simulink model "Single_phase_PF_measurement"  (R2024a)
settings: Solver=ode23  StartTime=0.0  StopTime=0.1  RelTol=1e-4
libraries: spsACVoltageSourceLib x3, spsCurrentMeasurementLib x3, spsPowerLib x3, spsSeriesRLCBranchLib x3, spsVoltageMeasurementLib x3, spspowerguiLib x3, spsRMSLib x2
settings Model: Creator=User  LastModifiedBy=User

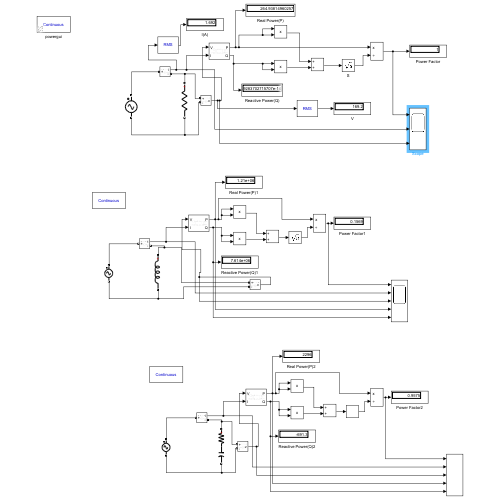
[thumbnail: Simulink's stored preview of the top-level diagram]
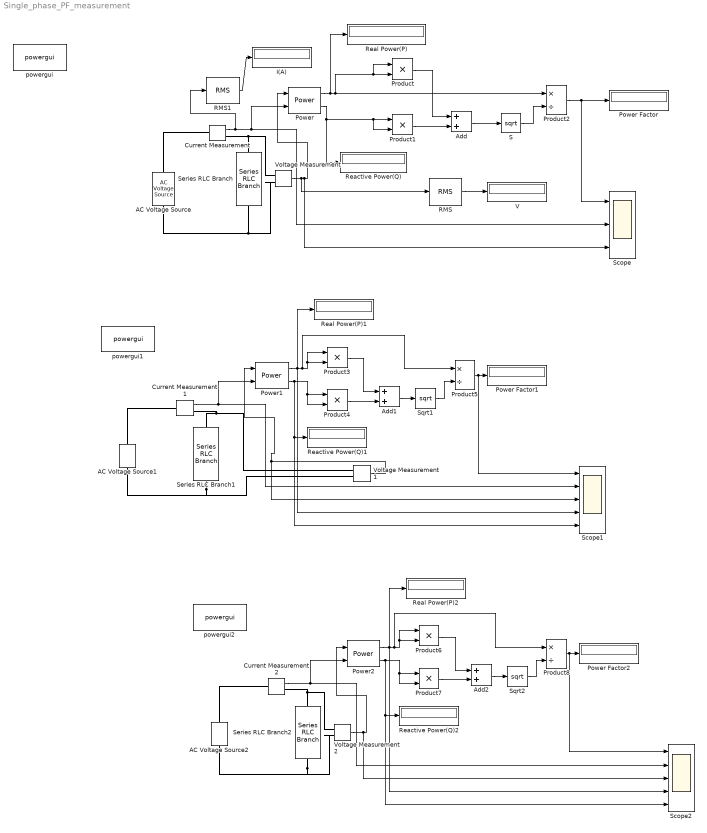
== system Single_phase_PF_measurement ==
  AC Voltage Source : spsACVoltageSourceLib/AC Voltage Source  Amplitude=230  Phase=0  Frequency=50  SampleTime=0  Measurements=None  BusType=swing  Pref=10e3  Qref=0  Qmin=-inf  Qmax=+inf
  AC Voltage Source1 : spsACVoltageSourceLib/AC Voltage Source  Amplitude=230  Phase=0  Frequency=50  SampleTime=0  Measurements=None  BusType=swing  Pref=10e3  Qref=0  Qmin=-inf  Qmax=+inf
  AC Voltage Source2 : spsACVoltageSourceLib/AC Voltage Source  Amplitude=230  Phase=0  Frequency=50  SampleTime=0  Measurements=None  BusType=swing  Pref=10e3  Qref=0  Qmin=-inf  Qmax=+inf
  Add : Sum
  Add1 : Sum
  Add2 : Sum
  Current Measurement : spsCurrentMeasurementLib/Current Measurement  PhasorSimulation=off  OutputType=Complex  PSBequivalent=0
  Current Measurement1 : spsCurrentMeasurementLib/Current Measurement  PhasorSimulation=off  OutputType=Complex  PSBequivalent=0
  Current Measurement2 : spsCurrentMeasurementLib/Current Measurement  PhasorSimulation=off  OutputType=Complex  PSBequivalent=0
  I(A) : Display
  Power : spsPowerLib/Power  Freq=60  Vinit=[1, 0]  Iinit=[1, 0]  Ts=0
  Power Factor : Display
  Power Factor1 : Display
  Power Factor2 : Display
  Power1 : spsPowerLib/Power  Freq=60  Vinit=[1, 0]  Iinit=[1, 0]  Ts=0
  Power2 : spsPowerLib/Power  Freq=60  Vinit=[1, 0]  Iinit=[1, 0]  Ts=0
  Product{,1,3..4,6..7} (6 alike) : Product
  Product2 : Product  Inputs=*/
  Product5 : Product  Inputs=*/
  Product8 : Product  Inputs=*/
  RMS : spsRMSLib/RMS  TrueRMS=on  Freq=60  RMSInit=120  Ts=0
  RMS1 : spsRMSLib/RMS  TrueRMS=on  Freq=60  RMSInit=120  Ts=0
  Reactive Power(Q) : Display
  Reactive Power(Q)1 : Display
  Reactive Power(Q)2 : Display
  Real Power(P) : Display
  Real Power(P)1 : Display
  Real Power(P)2 : Display
  S : Sqrt
  Scope : Scope  NumInputPorts=3
  Scope1 : Scope  NumInputPorts=5
  Scope2 : Scope  NumInputPorts=5
  Series RLC Branch : spsSeriesRLCBranchLib/Series RLC Branch  LConnTagsString=__new0  RConnTagsString=__new0  BranchType=R  Resistance=100  Inductance=1  SetiL0=off  InitialCurrent=0  Capacitance=40e-6  Setx0=off  InitialVoltage=0  Measurements=None
  Series RLC Branch1 : spsSeriesRLCBranchLib/Series RLC Branch  LConnTagsString=__new0  RConnTagsString=__new0  BranchType=L  Resistance=10  Inductance=10e-6  SetiL0=off  InitialCurrent=0  Capacitance=1e-6  Setx0=off  InitialVoltage=0  Measurements=None
  Series RLC Branch2 : spsSeriesRLCBranchLib/Series RLC Branch  LConnTagsString=__new0  RConnTagsString=__new0  BranchType=RC  Resistance=10  Inductance=10e-6  SetiL0=off  InitialCurrent=0  Capacitance=1e-3  Setx0=off  InitialVoltage=0  Measurements=None
  Sqrt1 : Sqrt
  Sqrt2 : Sqrt
  V : Display
  Voltage Measurement : spsVoltageMeasurementLib/Voltage Measurement  PhasorSimulation=off  OutputType=Complex  PSBequivalent=0
  Voltage Measurement1 : spsVoltageMeasurementLib/Voltage Measurement  PhasorSimulation=off  OutputType=Complex  PSBequivalent=0
  Voltage Measurement2 : spsVoltageMeasurementLib/Voltage Measurement  PhasorSimulation=off  OutputType=Complex  PSBequivalent=0
  powergui : spspowerguiLib/powergui  Priority=1  SimulationMode=Continuous  SampleTime=50e-6  frequency=60  Iterations=50  frequencyindice=50  Pbase=100e6  ErrMax=1e-4  UnitsV=kV  UnitsW=MW  buscounter=0  FunctionMessages=off  echomessages=off  EnableUseOfTLC=off  CurrentSourceSwitches=off  DisableSnubberDevices=off  DisableRonSwitches=off  DisableVfSwitches=off  DisplayEquations=off  AutomaticDiscreteSolvers=off  SolverType=Tustin/Backward Euler (TBE)  Interpol=off  ExternalGateDelay=off  methode=off  Ts=100  x0status=blocks  SPID=on  SwTol=0  HookPort=off  NonlinearTolerance=1e-4  nMaxIteration=100  ContinueOnMaxIteration=off  RestoreLinks=warning  ResistiveCurrentMeasurement=off  Frange=[0:2:500]  Ylog=off  Xlog=on  ShowGrid=off  save=off  variable=ZData  structure=0  ZoomFFT=off  StartTime=0.0  cycles=1  DisplayStyle=1  fundamental=60  FreqAxis=off  MaxFrequency=1000  frequencyindicesteady=1  RmsSteady=1  display=off
  powergui1 : spspowerguiLib/powergui  Priority=1  SimulationMode=Continuous  SampleTime=50e-6  frequency=60  Iterations=50  frequencyindice=50  Pbase=100e6  ErrMax=1e-4  UnitsV=kV  UnitsW=MW  buscounter=0  FunctionMessages=off  echomessages=off  EnableUseOfTLC=off  CurrentSourceSwitches=off  DisableSnubberDevices=off  DisableRonSwitches=off  DisableVfSwitches=off  DisplayEquations=off  AutomaticDiscreteSolvers=off  SolverType=Tustin/Backward Euler (TBE)  Interpol=off  ExternalGateDelay=off  methode=off  Ts=100  x0status=blocks  SPID=on  SwTol=0  HookPort=off  NonlinearTolerance=1e-4  nMaxIteration=100  ContinueOnMaxIteration=off  RestoreLinks=warning  ResistiveCurrentMeasurement=off  Frange=[0:2:500]  Ylog=off  Xlog=on  ShowGrid=off  save=off  variable=ZData  structure=0  ZoomFFT=off  StartTime=0.0  cycles=1  DisplayStyle=1  fundamental=60  FreqAxis=off  MaxFrequency=1000  frequencyindicesteady=1  RmsSteady=1  display=off
  powergui2 : spspowerguiLib/powergui  Priority=1  SimulationMode=Continuous  SampleTime=50e-6  frequency=60  Iterations=50  frequencyindice=50  Pbase=100e6  ErrMax=1e-4  UnitsV=kV  UnitsW=MW  buscounter=0  FunctionMessages=off  echomessages=off  EnableUseOfTLC=off  CurrentSourceSwitches=off  DisableSnubberDevices=off  DisableRonSwitches=off  DisableVfSwitches=off  DisplayEquations=off  AutomaticDiscreteSolvers=off  SolverType=Tustin/Backward Euler (TBE)  Interpol=off  ExternalGateDelay=off  methode=off  Ts=100  x0status=blocks  SPID=on  SwTol=0  HookPort=off  NonlinearTolerance=1e-4  nMaxIteration=100  ContinueOnMaxIteration=off  RestoreLinks=warning  ResistiveCurrentMeasurement=off  Frange=[0:2:500]  Ylog=off  Xlog=on  ShowGrid=off  save=off  variable=ZData  structure=0  ZoomFFT=off  StartTime=0.0  cycles=1  DisplayStyle=1  fundamental=60  FreqAxis=off  MaxFrequency=1000  frequencyindicesteady=1  RmsSteady=1  display=off
  wires:
  Voltage Measurement/1 -> RMS/1, Scope/3, Power/1
  Current Measurement/1 -> RMS1/1, Power/2, Scope/2
  Power/1 -> Real Power(P)/1, Product2/1, Product/2, Product/1
  Power/2 -> Reactive Power(Q)/1, Product1/2, Product1/1
  Add/1 -> S/1
  Product/1 -> Add/1
  Product1/1 -> Add/2
  S/1 -> Product2/2
  Product2/1 -> Scope/1, Power Factor/1
  Add1/1 -> Sqrt1/1
  Sqrt1/1 -> Product5/2
  Power1/2 -> Scope1/5, Reactive Power(Q)1/1, Product4/2, Product4/1
  Current Measurement1/1 -> Scope1/2, Power1/2
  Voltage Measurement1/1 -> Scope1/3, Power1/1
  Product5/1 -> Scope1/1, Power Factor1/1
  Product4/1 -> Add1/2
  Product3/1 -> Add1/1
  Power1/1 -> Scope1/4, Real Power(P)1/1, Product5/1, Product3/2, Product3/1
  Product7/1 -> Add2/2
  Product8/1 -> Scope2/1, Power Factor2/1
  Product6/1 -> Add2/1
  Voltage Measurement2/1 -> Scope2/3, Power2/1
  Power2/2 -> Scope2/5, Reactive Power(Q)2/1, Product7/2, Product7/1
  Current Measurement2/1 -> Power2/2, Scope2/2
  Power2/1 -> Real Power(P)2/1, Scope2/4, Product8/1, Product6/2, Product6/1
  Sqrt2/1 -> Product8/2
  Add2/1 -> Sqrt2/1
  RMS/1 -> V/1
  RMS1/1 -> I(A)/1
  connections:
  AC Voltage Source/RConn1 -- Current Measurement/LConn1
  Series RLC Branch/LConn1 -- Voltage Measurement/LConn1 -- Current Measurement/RConn1
  AC Voltage Source/LConn1 -- Series RLC Branch/RConn1 -- Voltage Measurement/LConn2
  Series RLC Branch1/LConn1 -- Voltage Measurement1/LConn1 -- Current Measurement1/RConn1
  Series RLC Branch1/RConn1 -- Voltage Measurement1/LConn2 -- AC Voltage Source1/LConn1
  AC Voltage Source1/RConn1 -- Current Measurement1/LConn1
  Series RLC Branch2/RConn1 -- AC Voltage Source2/LConn1 -- Voltage Measurement2/LConn2
  Series RLC Branch2/LConn1 -- Voltage Measurement2/LConn1 -- Current Measurement2/RConn1
  AC Voltage Source2/RConn1 -- Current Measurement2/LConn1
